simulink model "ControlSystemModel"  (R2021a)
settings: Solver=FixedStepAuto  StartTime=0.0  StopTime=20.0  FixedStep=sample_time  RelTol=1e-3
InitFcn:
  | clear,
  | SampleTime,
  | SystemParameters
settings Model: Creator=computador  LastModifiedBy=computador

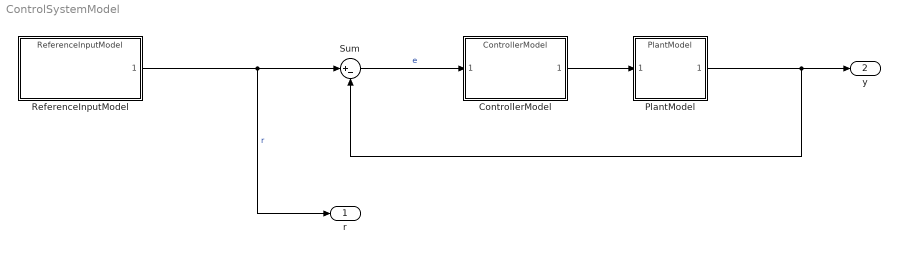
== system ControlSystemModel ==
  ControllerModel : ModelReference  ModelNameDialog=ControllerModel  SimulationMode=Normal  ModelReferenceVersion=1.11
  PlantModel : ModelReference  ModelNameDialog=PlantModel  SimulationMode=Normal  ModelReferenceVersion=1.11
  ReferenceInputModel : ModelReference  ModelNameDialog=ReferenceInputModel  SimulationMode=Normal  ModelReferenceVersion=1.12
  Sum : Sum  Inputs=|+-
  r : Outport
  y : Outport  Port=2
  wires:
  PlantModel/1 -> y/1, Sum/2
  Sum/1 -> ControllerModel/1  "e"
  ControllerModel/1 -> PlantModel/1
  ReferenceInputModel/1 -> r/1, Sum/1  "r"
